simulink model "Flap"  (R2023a)
settings: Solver=FixedStepAuto  StartTime=0.0  StopTime=Inf  RelTol=1e-3  SampleTimeConstraint=STIndependent
undefined symbols (not defined in the file): BIT_MASK_COINS_FLAP, BIT_MASK_COINS_FLAP_NOT, char2dec, PERIPHERALS_REGISTER
libraries: simulink x2
Description:
  | % Copyright 2023 The MathWorks, Inc.
settings Model: DataDictionary=Parameters.sldd  EnableAccessToBaseWorkspace=off  Creator=sdupertu  LastModifiedBy=sdupertu
settings SolverCC: AlgebraicLoopSolver=TrustRegion
settings DataIOCC: SaveOutput=off  SaveTime=off
settings OptimizationCC: DefaultParameterBehavior=Inlined  EnhancedBackFolding=on  PassReuseOutputArgsAs=Individual arguments  OptimizeBlockOrder=speed  DifferentSizesBufferReuse=on  OptimizationCustomize=off  EfficientTunableParamExpr=on
settings DebuggingCC: ParameterTunabilityLossMsg=error  UnconnectedInputMsg=warning  UnconnectedOutputMsg=warning  UnconnectedLineMsg=warning  PregeneratedLibrarySubsystemCodeDiagnostic=none  ArithmeticOperatorsInVariantConditions=warning
settings ModelReferenceCC: EnableRefExpFcnMdlSchedulingChecks=on  EnableParallelModelReferenceBuilds=on
settings SFSimCC: SimUseLocalCustomCode=off  MATLABDynamicMemAlloc=off  CustomCodeUndefinedFunction=UseInterfaceOnly
settings RTWCC: Description=Embedded Coder  SystemTargetFile=ert.tlc  TemplateMakefile=ert_default_tmf  RTWUseLocalCustomCode=off  IncludeHyperlinkInReport=on  DLArmComputeVersion=19.05
settings CodeAppCC: ForceParamTrailComments=on  IgnoreCustomStorageClasses=off  MaxIdLength=61  OperatorAnnotations=on  SimulinkDataObjDesc=on  SFDataObjDesc=on  InsertBlockDesc=on
settings ERTTargetCC: TargetLangStandard=C99 (ISO)  GenerateSampleERTMain=on  InlinedParameterPlacement=NonHierarchical  ERTCustomFileTemplate=example_file_process.tlc

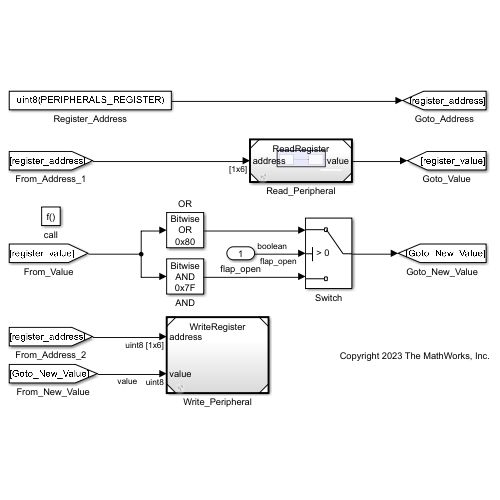
[thumbnail: Simulink's stored preview of the top-level diagram]
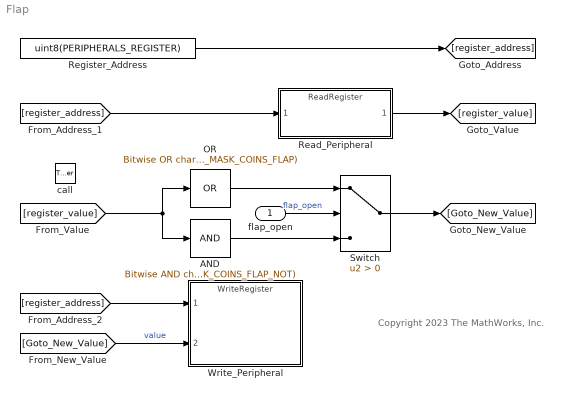
== system Flap ==
  note: Copyright 2023 The MathWorks, Inc.
  flap_open : Inport  OutDataTypeStr=boolean  PortDimensions=1
  call : TriggerPort  TriggerType=function-call  VariantControl=Variant  PortDimensions=1  TriggerSignalSampleTime=[0.001,0]
  AND : simulink/Logic and Bit Operations/Bitwise Operator  logicop=AND  UseBitMask=on  BitMask=char2dec(BIT_MASK_COINS_FLAP_NOT)  BitMaskRealWorld=Stored Integer
  OR : simulink/Logic and Bit Operations/Bitwise Operator  logicop=OR  UseBitMask=on  BitMask=char2dec(BIT_MASK_COINS_FLAP)  BitMaskRealWorld=Stored Integer
  Read_Peripheral : ModelReference  ModelNameDialog=ReadRegister  SimulationMode=Normal  ModelReferenceVersion=8.7
  Register_Address : Constant  Value=uint8(PERIPHERALS_REGISTER)  SampleTime=-1
  Switch : Switch  Criteria=u2 > Threshold  SaturateOnIntegerOverflow=off  InputSameDT=off
  Write_Peripheral : ModelReference  ModelNameDialog=WriteRegister  SimulationMode=Normal  ModelReferenceVersion=8.2
  wires:
  Register_Address/1 -> [register_address]
  [register_address] -> Write_Peripheral/1
  [register_address] -> Read_Peripheral/1
  Read_Peripheral/1 -> [register_value]
  flap_open/1 -> Switch/2  "flap_open"
  [register_value] -> AND/1, OR/1
  Switch/1 -> [Goto_New_Value]
  [Goto_New_Value] -> Write_Peripheral/2  "value"
  OR/1 -> Switch/1
  AND/1 -> Switch/3
